simulink model "complete_robot_sim"  (R2024b)
settings: Solver=FixedStepAuto  StartTime=0.0  StopTime=Tsim  FixedStep=1e-4  RelTol=1e-3
values from neighbouring files (symbols this model uses):
  g = 9.81    [complete_parameters.m]
  l = 0.08    [complete_parameters.m]
  m_b = 1    [complete_parameters.m]
  P = [m_b;m_w;l;g;r;d;Jw;Jbod]    [complete_parameters.m]
  r = 0.055    [complete_parameters.m]
  T_hold = 0.45    [complete_parameters.m]
  w_max = 20    [complete_parameters.m]
undefined symbols (not defined in the file or in its folder): Kp_t, Kp_v, Td_t, Td_v, Ti_t, Ti_v, X0
libraries: slpidlib x2, simulink x1
settings Model: Creator=jerem  LastModifiedBy=jerem

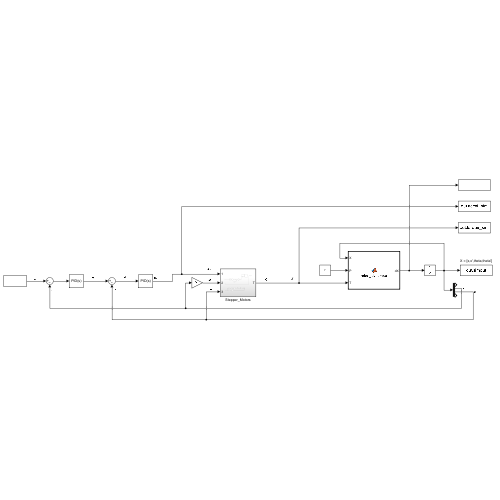
[thumbnail: Simulink's stored preview of the top-level diagram]
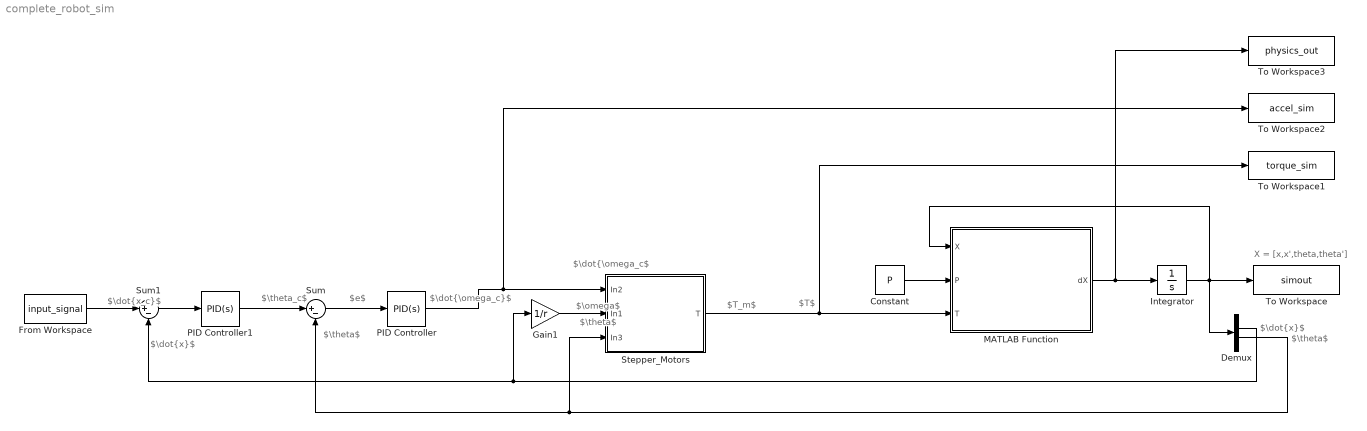
== system complete_robot_sim ==
  note: $\dot{\omega_c}$
  note: $\dot{x}$
  note: $\theta$
  note: $e$
  note: $\theta_c$
  note: X = [x,x',theta,theta']
  note: $\dot{x_c}$
  note: $T_m$
  note: $T$
  note: $\dot{\omega_c$
  note: $\omega$
  note: $\theta$
  note: $\dot{x}$
  note: $\theta$
  Constant : Constant  Value=P
  Demux : Demux
  From Workspace : FromWorkspace  VariableName=input_signal
  Gain1 : Gain  Gain=1/r
  Integrator : Integrator  InitialCondition=X0
  MATLAB Function : MATLAB Function  TreatAsAtomicUnit=on
  PID Controller : slpidlib/PID Controller  Controller=PID  Form=Parallel  TimeDomain=Continuous-time  UseExternalTs=off  SampleTime=-1  IntegratorMethod=Forward Euler  FilterMethod=Forward Euler  ControllerParametersSource=internal  P=Kp_t  I=Ti_t  UseKiTs=off  D=Td_t  UseExternalDerivativeSource=off  N=100  UseFilter=on  TunerSelectOption=Transfer Function Based (PID Tuner App)  InitialConditionSource=internal  InitialConditionForIntegrator=0  InitialConditionForFilter=0  DifferentiatorICPrevScaledInput=0  ExternalReset=none  TrackingMode=off  Kt=1  LimitOutput=off  SatLimitsSource=internal  UpperSaturationLimit=inf  LowerSaturationLimit=-inf  LinearizeAsGain=on  AntiWindupMode=none  Kb=1  LimitIntegrator=off  UpperIntegratorSaturationLimit=inf  LowerIntegratorSaturationLimit=-inf  POutMin=[]  POutMax=[]  IOutMin=[]  IOutMax=[]  DOutMin=[]  DOutMax=[]  NOutMin=[]  NOutMax=[]  SumOutMin=[]  SumOutMax=[]  SaturationOutMin=[]  SaturationOutMax=[]  PParamMin=[]  PParamMax=[]  IParamMin=[]  IParamMax=[]  DParamMin=[]  DParamMax=[]  NParamMin=[]  NParamMax=[]  KbParamMin=[]  KbParamMax=[]  KtParamMin=[]  KtParamMax=[]  KbOutMin=[]  KbOutMax=[]  KtOutMin=[]  KtOutMax=[]  IntegratorOutMin=[]  IntegratorOutMax=[]  FilterOutMin=[]  FilterOutMax=[]  SumI1OutMin=[]  SumI1OutMax=[]  SumI2OutMin=[]  SumI2OutMax=[]  SumI3OutMin=[]  SumI3OutMax=[]  SumI4OutMin=[]  SumI4OutMax=[]  SumDOutMin=[]  SumDOutMax=[]  DifferentiatorOutMin=[]  DifferentiatorOutMax=[]  FilterDiffOutCoefMin=[]  FilterDiffOutCoefMax=[]  ReciprocalOutMin=[]  ReciprocalOutMax=[]  SumDenOutMin=[]  SumDenOutMax=[]  SumNumOutMin=[]  SumNumOutMax=[]  DivideOutMin=[]  DivideOutMax=[]  UdiffTsProdOutMin=[]  UdiffTsProdOutMax=[]  NTsProdOutMin=[]  NTsProdOutMax=[]  UintegralTsProdOutMin=[]  UintegralTsProdOutMax=[]  UngainTsProdOutMin=[]  UngainTsProdOutMax=[]  ClampingZeroOutDataTypeStr=Inherit: Inherit via back propagation  ClampingZeroOutMin=[]  ClampingZeroOutMax=[]  FilterDenConstantOutDataTypeStr=Inherit: Inherit via back propagation  FilterDenConstantOutMin=[]  FilterDenConstantOutMax=[]  PCopyOutDataTypeStr=Inherit: Inherit via back propagation  PCopyOutMin=[]  PCopyOutMax=[]  NCopyOutDataTypeStr=Inherit: Inherit via back propagation  NCopyOutMin=[]  NCopyOutMax=[]  IntegratorContinuousStateAttributes=''  IntegratorStateMustResolveToSignalObject=off  IntegratorRTWStateStorageClass=Auto  FilterContinuousStateAttributes=''  FilterStateMustResolveToSignalObject=off  FilterRTWStateStorageClass=Auto  ParallelPVariant=InternalParameters  IdealPVariant=Disabled  IVariant=InternalParameters  DVariant=InternalParameters  IntegratorVariant=Continuous  SatVariant=Disabled  AWVariant=Passthrough  PCopyVariant=Disabled  TRVariant=Disabled  FdbkBlocksVariant=Forward  IdealPFdbkVariant=Disabled  SatFdbkVariant=Disabled  DerivativeFilterVariant=ContFilter  NVariant=InternalParameters  NCopyVariant=Disabled  FilterICVariant=InternalICsFilter  IntegratorICVariant=InternalICs  ExternalResetVariant=Disabled  TRSumVariant=Passthrough  SumFdbkVariant=Disabled  SumVariant=Sum_PID  TsampFilterVariant=InternalTs  TsampNgainVariant=Passthrough  TsampIntegralVariant=Disabled_SignalSpec  ExternalSaturationOutDataTypeStr=Inherit: Same as second input  DerivativeSourceVariant=ErrorSignal  PreIntVariant=InternalPreInt
  PID Controller1 : slpidlib/PID Controller  Controller=PID  Form=Parallel  TimeDomain=Continuous-time  UseExternalTs=off  SampleTime=-1  IntegratorMethod=Forward Euler  FilterMethod=Forward Euler  ControllerParametersSource=internal  P=Kp_v  I=Ti_v  UseKiTs=off  D=Td_v  UseExternalDerivativeSource=off  N=100  UseFilter=on  TunerSelectOption=Transfer Function Based (PID Tuner App)  InitialConditionSource=internal  InitialConditionForIntegrator=0  InitialConditionForFilter=0  DifferentiatorICPrevScaledInput=0  ExternalReset=none  TrackingMode=off  Kt=1  LimitOutput=off  SatLimitsSource=internal  UpperSaturationLimit=inf  LowerSaturationLimit=-inf  LinearizeAsGain=on  AntiWindupMode=none  Kb=1  LimitIntegrator=off  UpperIntegratorSaturationLimit=inf  LowerIntegratorSaturationLimit=-inf  POutMin=[]  POutMax=[]  IOutMin=[]  IOutMax=[]  DOutMin=[]  DOutMax=[]  NOutMin=[]  NOutMax=[]  SumOutMin=[]  SumOutMax=[]  SaturationOutMin=[]  SaturationOutMax=[]  PParamMin=[]  PParamMax=[]  IParamMin=[]  IParamMax=[]  DParamMin=[]  DParamMax=[]  NParamMin=[]  NParamMax=[]  KbParamMin=[]  KbParamMax=[]  KtParamMin=[]  KtParamMax=[]  KbOutMin=[]  KbOutMax=[]  KtOutMin=[]  KtOutMax=[]  IntegratorOutMin=[]  IntegratorOutMax=[]  FilterOutMin=[]  FilterOutMax=[]  SumI1OutMin=[]  SumI1OutMax=[]  SumI2OutMin=[]  SumI2OutMax=[]  SumI3OutMin=[]  SumI3OutMax=[]  SumI4OutMin=[]  SumI4OutMax=[]  SumDOutMin=[]  SumDOutMax=[]  DifferentiatorOutMin=[]  DifferentiatorOutMax=[]  FilterDiffOutCoefMin=[]  FilterDiffOutCoefMax=[]  ReciprocalOutMin=[]  ReciprocalOutMax=[]  SumDenOutMin=[]  SumDenOutMax=[]  SumNumOutMin=[]  SumNumOutMax=[]  DivideOutMin=[]  DivideOutMax=[]  UdiffTsProdOutMin=[]  UdiffTsProdOutMax=[]  NTsProdOutMin=[]  NTsProdOutMax=[]  UintegralTsProdOutMin=[]  UintegralTsProdOutMax=[]  UngainTsProdOutMin=[]  UngainTsProdOutMax=[]  ClampingZeroOutDataTypeStr=Inherit: Inherit via back propagation  ClampingZeroOutMin=[]  ClampingZeroOutMax=[]  FilterDenConstantOutDataTypeStr=Inherit: Inherit via back propagation  FilterDenConstantOutMin=[]  FilterDenConstantOutMax=[]  PCopyOutDataTypeStr=Inherit: Inherit via back propagation  PCopyOutMin=[]  PCopyOutMax=[]  NCopyOutDataTypeStr=Inherit: Inherit via back propagation  NCopyOutMin=[]  NCopyOutMax=[]  IntegratorContinuousStateAttributes=''  IntegratorStateMustResolveToSignalObject=off  IntegratorRTWStateStorageClass=Auto  FilterContinuousStateAttributes=''  FilterStateMustResolveToSignalObject=off  FilterRTWStateStorageClass=Auto  ParallelPVariant=InternalParameters  IdealPVariant=Disabled  IVariant=InternalParameters  DVariant=InternalParameters  IntegratorVariant=Continuous  SatVariant=Disabled  AWVariant=Passthrough  PCopyVariant=Disabled  TRVariant=Disabled  FdbkBlocksVariant=Forward  IdealPFdbkVariant=Disabled  SatFdbkVariant=Disabled  DerivativeFilterVariant=ContFilter  NVariant=InternalParameters  NCopyVariant=Disabled  FilterICVariant=InternalICsFilter  IntegratorICVariant=InternalICs  ExternalResetVariant=Disabled  TRSumVariant=Passthrough  SumFdbkVariant=Disabled  SumVariant=Sum_PID  TsampFilterVariant=InternalTs  TsampNgainVariant=Passthrough  TsampIntegralVariant=Disabled_SignalSpec  ExternalSaturationOutDataTypeStr=Inherit: Same as second input  DerivativeSourceVariant=ErrorSignal  PreIntVariant=InternalPreInt
  Stepper_Motors : Subsystem
  Sum : Sum  Inputs=|+-
  Sum1 : Sum  Inputs=|+-
  To Workspace : ToWorkspace  VariableName=simout  SaveFormat=Structure With Time  SampleTime=-1
  To Workspace1 : ToWorkspace  VariableName=torque_sim  SaveFormat=Structure With Time  SampleTime=-1
  To Workspace2 : ToWorkspace  VariableName=accel_sim  SaveFormat=Structure With Time  SampleTime=-1
  To Workspace3 : ToWorkspace  VariableName=physics_out  SaveFormat=Structure With Time  SampleTime=-1
  wires:
  Constant/1 -> MATLAB Function/2(P)
  MATLAB Function/1(dX) -> Integrator/1, To Workspace3/1
  Integrator/1 -> Demux/1, To Workspace/1, MATLAB Function/1(X)
  PID Controller1/1 -> Sum/1
  Sum/1 -> PID Controller/1
  Demux/2 -> Gain1/1, Sum1/2
  Sum1/1 -> PID Controller1/1
  From Workspace/1 -> Sum1/1
  Demux/3 -> Stepper_Motors/3(In3), Sum/2
  Stepper_Motors/1(T) -> MATLAB Function/3(T), To Workspace1/1
  Gain1/1 -> Stepper_Motors/2(In1)
  PID Controller/1 -> To Workspace2/1, Stepper_Motors/1(In2)

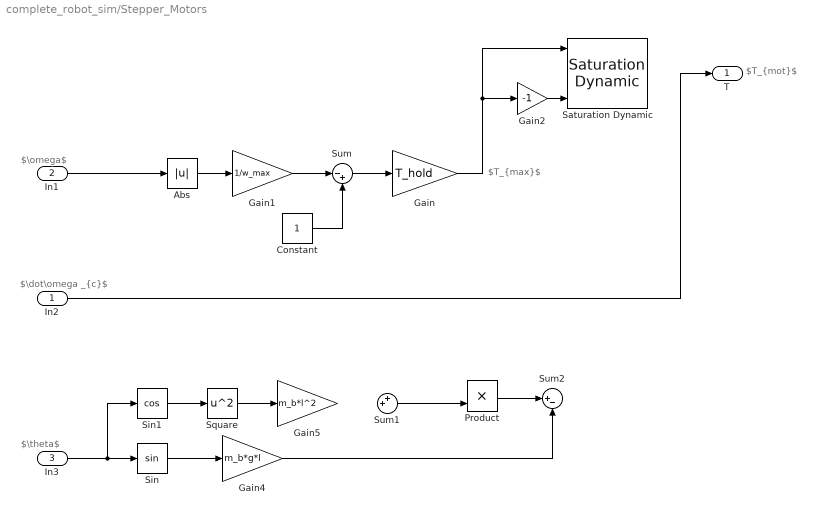
== system complete_robot_sim/Stepper_Motors ==
  note: $T_{max}$
  note: $\dot\omega _{c}$
  note: $T_{mot}$
  note: $\omega$
  note: $\theta$
  In2 : Inport
  In1 : Inport  Port=2
  In3 : Inport  Port=3
  Abs : Abs  SaturateOnIntegerOverflow=off
  Constant : Constant
  Gain : Gain  Gain=T_hold
  Gain1 : Gain  Gain=1/w_max
  Gain2 : Gain  Gain=-1
  Gain4 : Gain  Gain=m_b*g*l
  Gain5 : Gain  Gain=m_b*l^2
  Product : Product
  Saturation Dynamic : simulink/Discontinuities/Saturation Dynamic  OutMin=[]  OutMax=[]  OutDataTypeStr=Inherit: Same as second input  OutDataType=fixdt(1, 16)  OutScaling=2^-10  DoSatur=off
  Sin : Trigonometry
  Sin1 : Trigonometry  Operator=cos
  Square : Math  Operator=square
  Sum : Sum  Inputs=|-+
  Sum1 : Sum  Inputs=++|
  Sum2 : Sum  Inputs=|+-
  T : Outport
  wires:
  Constant/1 -> Sum/2
  Abs/1 -> Gain1/1
  Gain1/1 -> Sum/1
  Sum/1 -> Gain/1
  In1/1 -> Abs/1
  Gain2/1 -> Saturation Dynamic/3
  Gain/1 -> Saturation Dynamic/1, Gain2/1
  In3/1 -> Sin1/1, Sin/1
  Sin/1 -> Gain4/1
  Sin1/1 -> Square/1
  Square/1 -> Gain5/1
  Sum1/1 -> Product/2
  Product/1 -> Sum2/1
  Gain4/1 -> Sum2/2
  In2/1 -> T/1

== matlab function complete_robot_sim/MATLAB Function ==
  data: dX output; X input; P input; T input
function dX = robot_dynamics(X, P, T)
    % Compute robot dynamics based on the ODE's of movement
    % States
    x = X(1);
    x_dot = X(2);
    theta = X(3);
    theta_dot = X(4);
    
    % Parameters
    m_b = P(1);
    m_w = P(2);
    l = P(3);
    g = P(4);
    r = P(5);
    d = P(6);
    Jw = P(7);
    Jbod = P(8);
    
    % Define variables
    a = m_b*l;
    I_O = Jbod+m_b*l^2;
    m_tot=m_b+2*m_w;
    m_O=m_tot+Jw/r^2;
    d1=I_O*m_O-a^2*cos(theta)^2;

    % ODE's
    x_ddot = 1/d1*(a*I_O*theta_dot^2*sin(theta)...
             -a^2*g*sin(theta)*cos(theta)...
             +T*(I_O/r+a*cos(theta)));
    
    theta_ddot = 1/d1*(-a^2*theta_dot^2*sin(theta)*cos(theta) ...
                 +a*m_O*g*sin(theta)...
                 -T*(m_O+a/r*cos(theta)));
    
 
    % State derivatives
    dX = zeros(4,1);
    dX(1) = x_dot;
    dX(2) = x_ddot;
    dX(3) = theta_dot;
    dX(4) = theta_ddot;

end
